simulink model "FCTCR"  (R2013a)
settings: Solver=ode45  StartTime=0.0  StopTime=1  RelTol=1e-3
libraries: powerlib x13, powerlib_extras x5
settings Model: Creator=Anish Salavi  LastModifiedBy=Acer
settings DataIOCC: SignalLoggingSaveFormat=ModelDataLogs
settings OptimizationCC: ExpressionDepthLimit=2147483647
settings DebuggingCC: FcnCallInpInsideContextMsg=UseLocalSettings
settings GRTTargetCC: CombineOutputUpdateFcns=off  GRTInterface=on

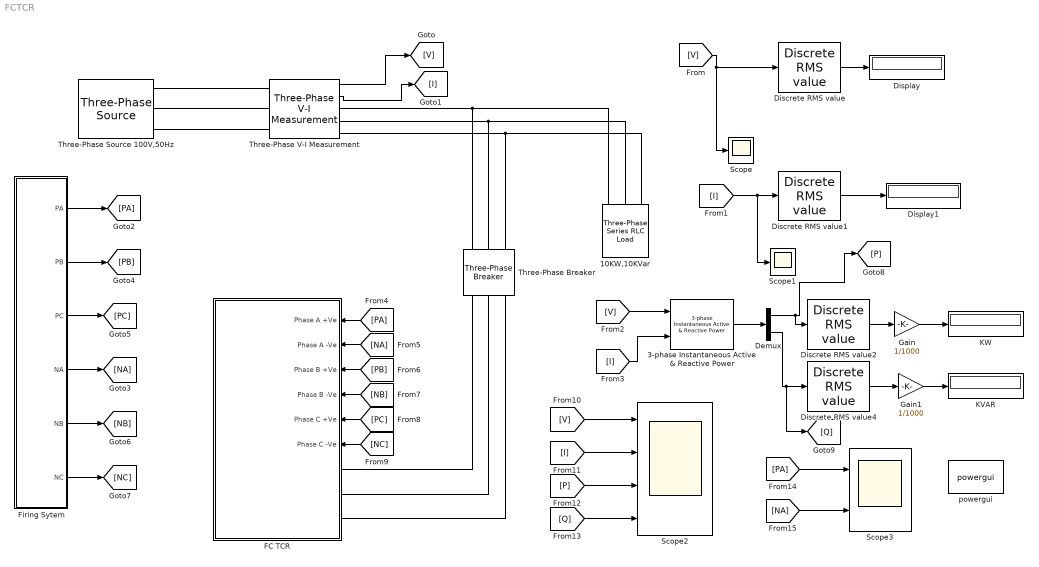
== system FCTCR ==
  10KW,10KVar : powerlib/Elements/Three-Phase Series RLC Load  LConnTagsString=A|B|C  Configuration=Y (grounded)  NominalVoltage=100  NominalFrequency=50  ActivePower=10e3  InductivePower=10e3  CapacitivePower=0  Measurements=None  LoadType=constant Z
  3-phase Instantaneous Active & Reactive Power : powerlib_extras/Measurements/3-phase  Instantaneous  Active & Reactive Power
  Demux : Demux  Outputs=2
  Discrete RMS value{,1..2,4} (4 alike) : powerlib_extras/Discrete Measurements/Discrete  RMS value  Freq=50  Mag_Init=0  Ts=50e-6
  Display : Display
  Display1 : Display
  FC TCR : Subsystem
  Firing Sytem : Subsystem
  Gain : Gain  Gain=1/1000
  Gain1 : Gain  Gain=1/1000
  KVAR : Display
  KW : Display
  Scope : Scope
      settings: YMin=-90  YMax=90
  Scope1 : Scope
  Scope2 : Scope  NumInputPorts=4
      settings: TimeRange=2.828919309205702e-005  YMin=-100~-100~0~-5000  YMax=100~200~20000~15000  SaveName=main
  Scope3 : Scope  NumInputPorts=2
      settings: TimeRange=5  YMin=0~0  YMax=20~20  SaveName=main1  SampleInput=on
  Three-Phase V-I Measurement : powerlib/Measurements/Three-Phase V-I Measurement  VoltageMeasurement=phase-to-ground  SetLabelV=off  LabelV=Vabc  Vpu=off  VpuLL=off  CurrentMeasurement=yes  SetLabelI=off  LabelI=Iabc  Ipu=off  Pbase=100e6  Vbase=500e3  OutputType=Complex  PhasorSimulation=off  PSBequivalent=0
  Three-Phase Breaker : powerlib/Elements/Three-Phase Breaker  InitialState=closed  SwitchA=on  SwitchB=on  SwitchC=on  SwitchTimes="[3/50  10/50]"  External=off  BreakerResistance=0.001  SnubberResistance=1e6  SnubberCapacitance=inf  Measurements=None
  Three-Phase Source 100V,50Hz : powerlib/Electrical Sources/Three-Phase Source  Voltage=100  PhaseAngle=0  Frequency=50  InternalConnection=Yn  SpecifyImpedance=off  Resistance=0  Inductance=0  ShortCircuitLevel=100e6  BaseVoltage=25e3  XRratio=7  BusType=swing  Pref=0  Qref=0  Qmin=-inf  Qmax=inf
  powergui : powerlib/powergui  Priority=1  SimulationMode=Discrete  SolverType=Tustin  SampleTime=50e-6  frequency=60  SPID=off  DisableSnubberDevices=off  DisableRonSwitches=off  DisableVfSwitches=off  SwTol=0  Interpol=off  DisplayEquations=off  frequencyindice=50  Pbase=100e6  ErrMax=1e-4  Iterations=50  UnitsV=kV  UnitsW=MW  FunctionMessages=off  echomessages=off  HookPort=off  EnableUseOfTLC=off  x0status=blocks  RestoreLinks=warning  ResistiveCurrentMeasurement=off  Frange=[0:2:500]  Ylog=off  Xlog=on  ShowGrid=off  save=off  variable=ZData  structure=main  ZoomFFT=off  StartTime=4.8  cycles=2  DisplayStyle=1  fundamental=50  FreqAxis=off  MaxFrequency=1000  frequencyindicesteady=1  RmsSteady=1  display=off  Ts=0  methode=off
  wires:
  Discrete RMS value/1 -> Display/1
  Three-Phase V-I Measurement/1 -> [V]
  Three-Phase V-I Measurement/2 -> [I]
  [V] -> Discrete RMS value/1, Scope/1
  [I] -> Discrete RMS value1/1, Scope1/1
  Discrete RMS value1/1 -> Display1/1
  [V] -> 3-phase Instantaneous Active & Reactive Power/1
  [I] -> 3-phase Instantaneous Active & Reactive Power/2
  3-phase Instantaneous Active & Reactive Power/1 -> Demux/1
  Demux/1 -> [P], Discrete RMS value2/1
  Gain/1 -> KW/1
  Gain1/1 -> KVAR/1
  [V] -> Scope2/1
  [I] -> Scope2/2
  [P] -> Scope2/3
  [Q] -> Scope2/4
  [PA] -> Scope3/1
  [NA] -> Scope3/2
  Firing Sytem/2(PB) -> [PB]
  Firing Sytem/3(PC) -> [PC]
  Firing Sytem/5(NB) -> [NB]
  Firing Sytem/4(NA) -> [NA]
  [PA] -> FC TCR/1(Phase A +Ve)
  [NA] -> FC TCR/2(Phase A -Ve)
  [NB] -> FC TCR/4(Phase B -Ve)
  [PB] -> FC TCR/3(Phase B +Ve)
  [PC] -> FC TCR/5(Phase C +Ve)
  [NC] -> FC TCR/6(Phase C -Ve)
  Firing Sytem/6(NC) -> [NC]
  Firing Sytem/1(PA) -> [PA]
  Discrete RMS value2/1 -> Gain/1
  Demux/2 -> Discrete RMS value4/1, [Q]
  Discrete RMS value4/1 -> Gain1/1
  connections:
  Three-Phase V-I Measurement/LConn1 -- Three-Phase Source 100V,50Hz/RConn1
  Three-Phase Source 100V,50Hz/RConn2 -- Three-Phase V-I Measurement/LConn2
  Three-Phase Source 100V,50Hz/RConn3 -- Three-Phase V-I Measurement/LConn3
  10KW,10KVar/LConn1 -- Three-Phase V-I Measurement/RConn1 -- Three-Phase Breaker/RConn1
  Three-Phase V-I Measurement/RConn2 -- Three-Phase Breaker/RConn2 -- 10KW,10KVar/LConn2
  Three-Phase V-I Measurement/RConn3 -- 10KW,10KVar/LConn3 -- Three-Phase Breaker/RConn3
  Three-Phase Breaker/LConn1 -- FC TCR/LConn1
  Three-Phase Breaker/LConn2 -- FC TCR/LConn2
  Three-Phase Breaker/LConn3 -- FC TCR/LConn3

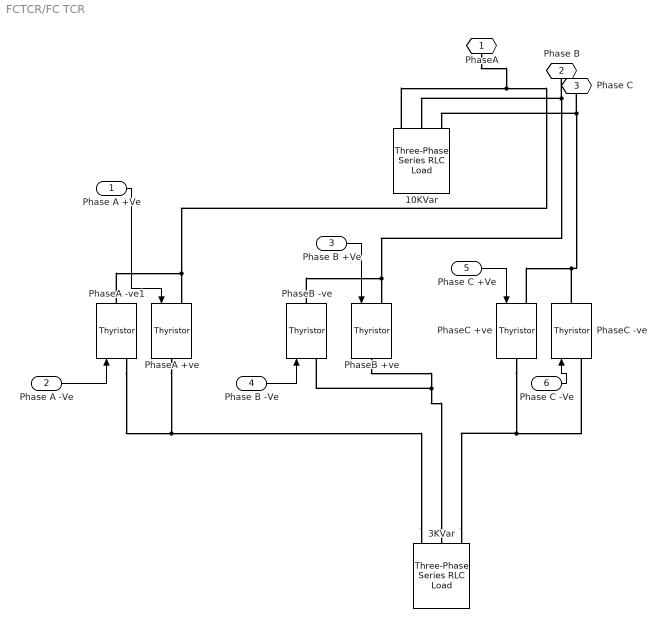
== system FCTCR/FC TCR ==
  Phase A +Ve : Inport
  Phase A -Ve : Inport  Port=2
  Phase B +Ve : Inport  Port=3
  Phase B -Ve : Inport  Port=4
  Phase C +Ve : Inport  Port=5
  Phase C -Ve : Inport  Port=6
  10KVar : powerlib/Elements/Three-Phase Series RLC Load  LConnTagsString=A|B|C  Configuration=Y (grounded)  NominalVoltage=100  NominalFrequency=50  ActivePower=1e-6  InductivePower=0  CapacitivePower=10e3  Measurements=None  LoadType=constant Z
  3KVar : powerlib/Elements/Three-Phase Series RLC Load  LConnTagsString=A|B|C  Configuration=Y (grounded)  NominalVoltage=100  NominalFrequency=50  ActivePower=0  InductivePower=3e3  CapacitivePower=0  Measurements=None  LoadType=constant Z
  PhaseA +ve : powerlib/Power Electronics/Thyristor  Ron=0.001  Lon=0  Vf=0.8  IC=0  Rs=500  Cs=250e-9  Measurements=off
  PhaseA -ve1 : powerlib/Power Electronics/Thyristor  Ron=0.001  Lon=0  Vf=0.8  IC=0  Rs=500  Cs=250e-9  Measurements=off
  PhaseB +ve : powerlib/Power Electronics/Thyristor  Ron=0.001  Lon=0  Vf=0.8  IC=0  Rs=500  Cs=250e-9  Measurements=off
  PhaseB -ve : powerlib/Power Electronics/Thyristor  Ron=0.001  Lon=0  Vf=0.8  IC=0  Rs=500  Cs=250e-9  Measurements=off
  PhaseC +ve : powerlib/Power Electronics/Thyristor  Ron=0.001  Lon=0  Vf=0.8  IC=0  Rs=500  Cs=250e-9  Measurements=off
  PhaseC -ve : powerlib/Power Electronics/Thyristor  Ron=0.001  Lon=0  Vf=0.8  IC=0  Rs=500  Cs=250e-9  Measurements=off
  PhaseA : PMIOPort  Port=1  Side=Left
  Phase B : PMIOPort  Port=2  Side=Left
  Phase C : PMIOPort  Port=3  Side=Left
  wires:
  Phase A +Ve/1 -> PhaseA +ve/1
  Phase A -Ve/1 -> PhaseA -ve1/1
  Phase B +Ve/1 -> PhaseB +ve/1
  Phase B -Ve/1 -> PhaseB -ve/1
  Phase C +Ve/1 -> PhaseC +ve/1
  Phase C -Ve/1 -> PhaseC -ve/1
  connections:
  3KVar/LConn1 -- PhaseA -ve1/LConn1 -- PhaseA +ve/RConn1
  3KVar/LConn2 -- PhaseB +ve/RConn1 -- PhaseB -ve/LConn1
  3KVar/LConn3 -- PhaseC +ve/RConn1 -- PhaseC -ve/LConn1
  10KVar/LConn1 -- PhaseA -ve1/RConn1 -- PhaseA +ve/LConn1 -- PhaseA/RConn1
  Phase B/RConn1 -- PhaseB +ve/LConn1 -- PhaseB -ve/RConn1 -- 10KVar/LConn2
  Phase C/RConn1 -- PhaseC +ve/LConn1 -- PhaseC -ve/RConn1 -- 10KVar/LConn3

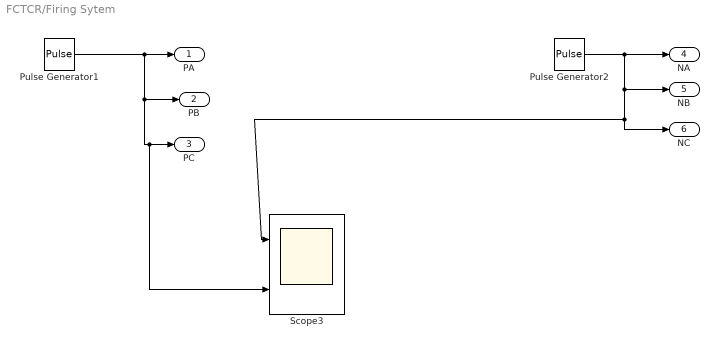
== system FCTCR/Firing Sytem ==
  Pulse Generator1 : DiscretePulseGenerator  PulseType=Time based  Amplitude=10  Period=0.02  PulseWidth=20  PhaseDelay=2.222e-3  VectorParams1D=off
  Pulse Generator2 : DiscretePulseGenerator  PulseType=Time based  Amplitude=10  Period=0.02  PulseWidth=20  PhaseDelay=2.2222e-3  VectorParams1D=off
  Scope3 : Scope  NumInputPorts=2
      settings: TimeRange=0.1  YMin=0~0  YMax=1~10  SaveName=main2
  PA : Outport
  PB : Outport  Port=2
  PC : Outport  Port=3
  NA : Outport  Port=4
  NB : Outport  Port=5
  NC : Outport  Port=6
  wires:
  Pulse Generator1/1 -> PA/1, PB/1, PC/1, Scope3/2
  Pulse Generator2/1 -> NA/1, NB/1, NC/1, Scope3/1
